simulink model "Relay_Auto_Tuning"  (R2017a)
settings: Solver=FixedStepAuto  StartTime=0  StopTime=1000  FixedStep=0.1  MaxStep=1e-1  MinStep=1e-2  RelTol=1e-3
values from neighbouring files (symbols this model uses):
  TF = tf(G)    [Relay_Identification.m]
settings Model: Creator=juliu  LastModifiedBy=juliu

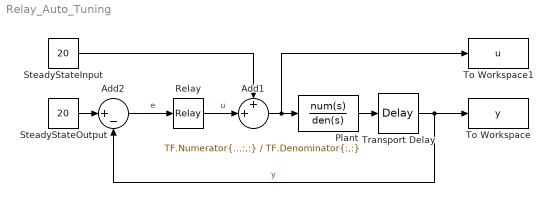
== system Relay_Auto_Tuning ==
  Add1 : Sum  Inputs=++|
  Add2 : Sum  Inputs=|+-
  Plant : TransferFcn  Numerator=TF.Numerator{:,:}  Denominator=TF.Denominator{:,:}
  Relay : Relay  OnSwitchValue=1  OffSwitchValue=-1  OnOutputValue=10  OffOutputValue=-3
  SteadyStateInput : Constant  Value=20
  SteadyStateOutput : Constant  Value=20
  To Workspace : ToWorkspace  VariableName=y  SaveFormat=Timeseries  SampleTime=-1
  To Workspace1 : ToWorkspace  VariableName=u  SaveFormat=Timeseries  SampleTime=-1
  Transport Delay : TransportDelay  DelayTime=0  InitialOutput=20
  wires:
  Plant/1 -> Transport Delay/1
  Relay/1 -> Add1/2  "u"
  SteadyStateInput/1 -> Add1/1
  Add1/1 -> To Workspace1/1, Plant/1
  Transport Delay/1 -> Add2/2, To Workspace/1  "y"
  Add2/1 -> Relay/1  "e"
  SteadyStateOutput/1 -> Add2/1
